simulink library "CDS_PARTS"  (Simulink 7.2)
settings: Solver=ode45  SolverMode=SingleTasking  StartTime=0.0  StopTime=10.0  RelTol=1e-3
undefined symbols (not defined in the file): dac, Subsystem
libraries: CDS_PARTS x5, simulink x2, cdsEXC x1, cdsEpicsBinIn x1, cdsEpicsIn x1, cdsEpicsMomentary x1, cdsEpicsOut x1, cdsRemoteIntlk x1, cdsEzCaRead x1, cdsEzCaWrite x1, cdsFiltCtrl x1, cdsFilt x1
settings Model: Creator=aivanov  LastModifiedBy=rolf  ExtModeAutoUpdateStatusClock=off

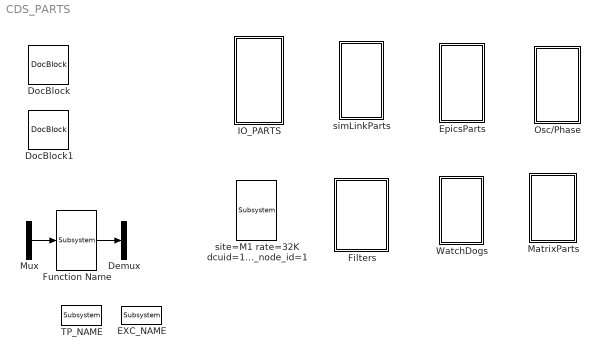
== system CDS_PARTS ==
  Demux : Demux  Outputs=2
  DocBlock : simulink/Model-Wide Utilities/DocBlock  Tag=Overview  SystemSampleTime=-1  DocumentType=Text
      settings: AttributesFormatString=%<Tag>
  DocBlock1 : simulink/Model-Wide Utilities/DocBlock  Tag=SW Install  SystemSampleTime=-1  DocumentType=Text
      settings: AttributesFormatString=%<Tag>
  EXC_NAME : cdsEXC/Subsystem  Tag=Excitation  SystemSampleTime=-1
      settings: AttributesFormatString=%<Tag>
  EpicsParts : Subsystem
  Filters : Subsystem
  Function Name : cdsFunctionCall/Subsystem  Tag=cdsFunctionCall  Description=|  SystemSampleTime=-1
      | Allows to make a call to external C function from the front-end code.                                                                                        
      | User needs to use a Mux and a Demux to proved N number of inputs and M number of outputs to an external function.                                            
      | Function "Foo()" code needs to be put in a file Foo.c in advLigo/src/fe/<model> directory.                                                                   
      |                                                                                                                                                              
      | Mon Apr  6 15:31:59 PDT 2009, by aivanov                                                                                                                     
      | It is possible now to put the same code you would normally keep in a file right here in this Description text box. The very first line needs to be 8 symbols:
      | //inline                                                                                                                                                     
      |                                                                                                                                                              
      | Then function definition follows exactly like you would put it in a file mentioned above.
      settings: AttributesFormatString=%<Tag>
  IO_PARTS : Subsystem
  MatrixParts : Subsystem
  Mux : Mux  Inputs=2
  Osc/Phase : Subsystem
  TP_NAME : cdsTP/Subsystem  Tag=Test Point  SystemSampleTime=-1
      settings: AttributesFormatString=%<Tag>
  WatchDogs : Subsystem
  simLinkParts : Subsystem
  site=M1 rate=32K dcuid=10 gds_node_id=1 : cdsParameters/Subsystem  Tag=cdsParameters  Description=|  SystemSampleTime=-1
      | Purpose:                                                                                                                                                                                                                                
      | Provide system parameters to the FE code generator to properly configure the generated EPICS names, rep rate of the FE controller, and the Data Acquisition node ID for proper storage of data from this FE controller.                 
      |                                                                                                                                                                                                                                         
      | Useage:                                                                                                                                                                                                                                 
      | The part NAME field is used to identify the FE parameters. It must be of the form:                                                                                                                                                      
      | site=                                                                                                                                                                                                                                   
      | rate=                                                                                                                                                                                                                                   
      | dcuid=                                                                                                                                                                                                                                  
      |                                                                                                                                                                                                                                         
      | Where:                                                                                                                                                                                                                                  
      | site= argument may be H1, H2, L1, M1, G1, either as a single argument or multiple, for example site=H1,H2. These are the only names allowed. These will become the first two characters of all EPICS and signal names (for example G1:).
      |                                                                                                                                                                                                                                         
      | rate= may be 2K, 16K, 32K, or 64K                                                                                                                                                                                                       
      |                                                                                                                                                                                                                                         
      | dcuid= is site specific ie it must be unique at each site.
      settings: AttributesFormatString=%<Tag>
  wires:
  Function Name/1 -> Demux/1
  Mux/1 -> Function Name/1

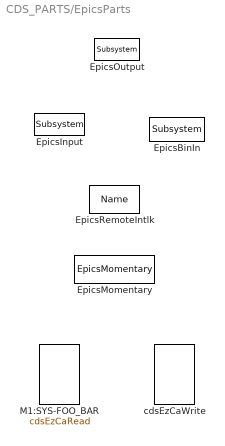
== system CDS_PARTS/EpicsParts ==
  EpicsBinIn : cdsEpicsBinIn/Subsystem  Tag=cdsEpicsBinIn  Description=|  SystemSampleTime=-1
      | Purpose:                                                                            
      | Create an EPICS binary (0 or 1) input channel to the FE realtime controls.          
      |                                                                                     
      | Operation:                                                                          
      | Outputs value from an EPICS ai record. Value is binary input (bi Epics record type).
      |                                                                                     
      | Usage:                                                                              
      | Name the part with the desired EPICS channel name.
      settings: AttributesFormatString=%<Tag>
  EpicsInput : cdsEpicsIn/Subsystem  Tag=cdsEpicsIn  Description=|  SystemSampleTime=-1
      | Purpose:                                                                              
      | Create an EPICS input channel connection to the FE realtime controls.                 
      |                                                                                       
      | Operation:                                                                            
      | Outputs value from an EPICS ai record. Value is floating point with a precision of 3..
      |                                                                                       
      | Usage:                                                                                
      | Name the part with the desired EPICS channel name.
      settings: AttributesFormatString=%<Tag>
  EpicsMomentary : cdsEpicsMomentary/EpicsMomentary  Tag=cdsEpicsMomentary  SystemSampleTime=-1
      settings: AttributesFormatString=%<Tag>
  EpicsOutput : cdsEpicsOut/Subsystem  Tag=cdsEpicsOutput  Description=|  SystemSampleTime=-1
      | Purpose:                                          
      | Output a FE signal to an EPICS channel.           
      |                                                   
      | Operation:                                        
      | Takes input value and passes it to EPICS record.  
      |                                                   
      | Usage:                                            
      | Name the part with the desired EPICS rrecord name.
      settings: AttributesFormatString=%<Tag>
  EpicsRemoteIntlk : cdsRemoteIntlk/Name  Tag=cdsRemoteIntlk  Description=|  SystemSampleTime=-1
      | Purpose:                                                                                                                                                                                                                                                                            
      | Used to turn off a switch in another subsystem using EPICS channel access. Typically, this is used as a remote interlock function.                                                                                                                                                  
      |                                                                                                                                                                                                                                                                                     
      | Operation:                                                                                                                                                                                                                                                                          
      | If input is zero, sends a zero to the specified EPICS channel name. Any other input value results in a NOOP. Input must be an integer.                                                                                                                                              
      |                                                                                                                                                                                                                                                                                     
      | Usage: Give the name of the EPICS channel to be written to, including the subsystem. For example: SEI-HMY_ACT_SW. This function will also produce a local EPICS variable for monitoring. For example, the above would result in a local EPICS variable of IFO:SUBSYS-SEI_HMY_ACT_SW.
      settings: AttributesFormatString=%<Tag>
  M1:SYS-FOO_BAR : cdsEzCaRead/cdsEzCaRead  Tag=cdsEzCaRead  Description=|  SystemSampleTime=-1
      | Purpose:                                                       
      | Used to input an Epics signal.                                 
      |                                                                
      | Operation:                                                     
      | Using ezcaread() function to get Epics input from a remote IOC.
      |                                                                
      | Usage:                                                         
      | Give the name of the EPICS channel to be read.
      settings: AttributesFormatString=%<Tag>
  cdsEzCaWrite : cdsEzCaWrite/cdsEzCaWrite  Tag=cdsEzCaWrite  Description=|  SystemSampleTime=-1
      | Purpose:                                    
      | Output Epics channel.                       
      |                                             
      | Operation:                                  
      | Using ezcawrite() output an Epics channel.  
      |                                             
      | Usage:                                      
      | Give the name of the EPICS channel to write.
      settings: AttributesFormatString=%<Tag>

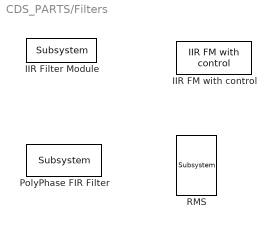
== system CDS_PARTS/Filters ==
  IIR FM with control : cdsFiltCtrl/IIR FM with control  Tag=cdsFiltCtrl  Description=|  SystemSampleTime=-1
      | cdsFiltCntrl is the standard IIR filter module (exactly the same as cdsFilt) but with added control data output 'Ctrl'. Filter module digital signal output appears on the first output, which is called 'Val'. 'Ctrl' output has a bit pattern encoding the state of filter's on/off switches (FM1 through FM10). The bit values are:
      |                                                                                                                                                                                                                                                                                                                                       
      | module 	hex	dec                                                                                                                                                                                                                                                                                                                       
      | -----------------------                                                                                                                                                                                                                                                                                                               
      | FM1	0x20                    32                                                                                                                                                                                                                                                                                                        
      | FM2	0x80                     128                                                                                                                                                                                                                                                                                                      
      | FM3	0x200                   512                                                                                                                                                                                                                                                                                                       
      | FM4	0x800                   2048                                                                                                                                                                                                                                                                                                      
      | FM5	0x2000                 8192                                                                                                                                                                                                                                                                                                       
      | FM6	0x8000                 32768                                                                                                                                                                                                                                                                                                      
      | FM7	0x20000                131072                                                                                                                                                                                                                                                                                                     
      | FM8	0x80000                 524288                                                                                                                                                                                                                                                                                                    
      | FM9	0x200000               2097152                                                                                                                                                                                                                                                                                                    
      | FM10	0x800000               8388608                                                                                                                                                                                                                                                                                                   
      |                                                                                                                                                                                                                                                                                                                                       
      | This bit data can be used to drive some other switches or it can be output using a binary I/O module.
      settings: AttributesFormatString=%<Tag>
  IIR Filter Module : cdsFilt/Subsystem  Tag=cdsFilt  Description=|  SystemSampleTime=-1
      | Purpose:                                                                                                                                                                                                                                  
      | Standard CDS IIR filter module.                                                                                                                                                                                                           
      |                                                                                                                                                                                                                                           
      | Operation:                                                                                                                                                                                                                                
      | Consists of 10 second order section IIR filters, plus a ramped gain stage. In FE code, also provides pre-defined test points and excitation channel inputs. The filter coefficients are defined in the LIGO system using the 'foton' tool.
      |                                                                                                                                                                                                                                           
      | Usage:                                                                                                                                                                                                                                    
      | Name the part with the desired filter module name.
      settings: AttributesFormatString=%<Tag>
  PolyPhase FIR Filter : cdsPPFIR/Subsystem  Tag=cdsPPFIR  Description=|  SystemSampleTime=-1
      | Purpose:                                                                                                    
      | Provide a Polyphase FIR filter algorithm. This part is typically only used in HEPI or other seismic systems.
      settings: AttributesFormatString=%<Tag>
  RMS : cdsRms/Subsystem  Tag=cdsRms  Description=|  SystemSampleTime=-1
      | Purpose:
      | Calculate an RMS based on the input signal.
      settings: AttributesFormatString=%<Tag>

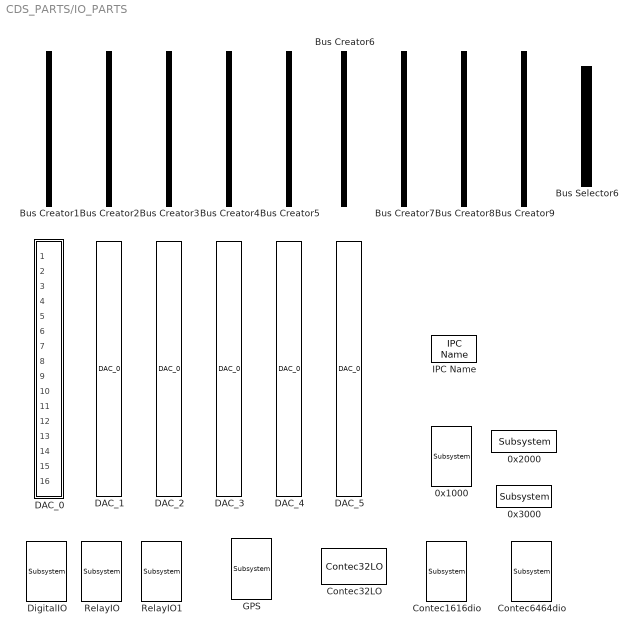
== system CDS_PARTS/IO_PARTS ==
  0x1000 : cdsRfmIO/Subsystem  Tag=cdsRfmIO  Description=VMIC5565 Reflective Memory read/write  SystemSampleTime=-1
      settings: AttributesFormatString=%<Tag>
  0x2000 : cdsIPC/Subsystem  Tag=cdsIPC  Description=Inter-process communication through /rtl_epics_ipc shared memory  SystemSampleTime=-1
      settings: AttributesFormatString=%<Tag>
  0x3000 : cdsIPCS/Subsystem  Tag=cdsIPCS  SystemSampleTime=-1
      settings: AttributesFormatString=%<Tag>
  Bus Creator1 : BusCreator  Tag=adc_0  Description=|  Inputs='adc_0_0','adc_0_1','adc_0_2','adc_0_3','adc_0_4','adc_0_5','adc_0_6','adc_0_7','adc_0_8','adc_0_9','adc_0_10','adc_0_11','adc_0_12','adc_0_13','adc_0_14','adc_0_15','adc_0_16','adc_0_17','adc_0_18','adc_0_19','adc_0_20','adc_0_21','adc_0_22','adc_0_23','adc_0_24','adc_0_25','adc_0_26','adc_0_27','adc_0_28','adc_0_29','adc_0_30','adc_0_31'
      | ADC0      
      | card_num=0
      settings: AttributesFormatString=%<Description>
  Bus Creator2 : BusCreator  Description=|  Inputs='adc_1_0','adc_1_1','adc_1_2','adc_1_3','adc_1_4','adc_1_5','adc_1_6','adc_1_7','adc_1_8','adc_1_9','adc_1_10','adc_1_11','adc_1_12','adc_1_13','adc_1_14','adc_1_15','adc_1_16','adc_1_17','adc_1_18','adc_1_19','adc_1_20','adc_1_21','adc_1_22','adc_1_23','adc_1_24','adc_1_25','adc_1_26','adc_1_27','adc_1_28','adc_1_29','adc_1_30','adc_1_31'
      | ADC1      
      | card_num=1
      settings: AttributesFormatString=%<Description>
  Bus Creator3 : BusCreator  Description=|  Inputs='adc_2_0','adc_2_1','adc_2_2','adc_2_3','adc_2_4','adc_2_5','adc_2_6','adc_2_7','adc_2_8','adc_2_9','adc_2_10','adc_2_11','adc_2_12','adc_2_13','adc_2_14','adc_2_15','adc_2_16','adc_2_17','adc_2_18','adc_2_19','adc_2_20','adc_2_21','adc_2_22','adc_2_23','adc_2_24','adc_2_25','adc_2_26','adc_2_27','adc_2_28','adc_2_29','adc_2_30','adc_2_31'
      | ADC2      
      | card_num=2
      settings: AttributesFormatString=%<Description>
  Bus Creator4 : BusCreator  Description=|  Inputs='adc_3_0','adc_3_1','adc_3_2','adc_3_3','adc_3_4','adc_3_5','adc_3_6','adc_3_7','adc_3_8','adc_3_9','adc_3_10','adc_3_11','adc_3_12','adc_3_13','adc_3_14','adc_3_15','adc_3_16','adc_3_17','adc_3_18','adc_3_19','adc_3_20','adc_3_21','adc_3_22','adc_3_23','adc_3_24','adc_3_25','adc_3_26','adc_3_27','adc_3_28','adc_3_29','adc_3_30','adc_3_31'
      | ADC3      
      | card_num=3
      settings: AttributesFormatString=%<Description>
  Bus Creator5 : BusCreator  Description=|  Inputs='adc_4_0','adc_4_1','adc_4_2','adc_4_3','adc_4_4','adc_4_5','adc_4_6','adc_4_7','adc_4_8','adc_4_9','adc_4_10','adc_4_11','adc_4_12','adc_4_13','adc_4_14','adc_4_15','adc_4_16','adc_4_17','adc_4_18','adc_4_19','adc_4_20','adc_4_21','adc_4_22','adc_4_23','adc_4_24','adc_4_25','adc_4_26','adc_4_27','adc_4_28','adc_4_29','adc_4_30','adc_4_31'
      | ADC4      
      | card_num=4
      settings: AttributesFormatString=%<Description>
  Bus Creator6 : BusCreator  Description=|  Inputs='adc_5_0','adc_5_1','adc_5_2','adc_5_3','adc_5_4','adc_5_5','adc_5_6','adc_5_7','adc_5_8','adc_5_9','adc_5_10','adc_5_11','adc_5_12','adc_5_13','adc_5_14','adc_5_15','adc_5_16','adc_5_17','adc_5_18','adc_5_19','adc_5_20','adc_5_21','adc_5_22','adc_5_23','adc_5_24','adc_5_25','adc_5_26','adc_5_27','adc_5_28','adc_5_29','adc_5_30','adc_5_31'
      | ADC5      
      | card_num=5
      settings: AttributesFormatString=%<Description>
  Bus Creator7 : BusCreator  Description=|  Inputs='adc_6_0','adc_6_1','adc_6_2','adc_6_3','adc_6_4','adc_6_5','adc_6_6','adc_6_7','adc_6_8','adc_6_9','adc_6_10','adc_6_11','adc_6_12','adc_6_13','adc_6_14','adc_6_15','adc_6_16','adc_6_17','adc_6_18','adc_6_19','adc_6_20','adc_6_21','adc_6_22','adc_6_23','adc_6_24','adc_6_25','adc_6_26','adc_6_27','adc_6_28','adc_6_29','adc_6_30','adc_6_31'
      | ADC6      
      | card_num=6
      settings: AttributesFormatString=%<Description>
  Bus Creator8 : BusCreator  Description=|  Inputs='adc_7_0','adc_7_1','adc_7_2','adc_7_3','adc_7_4','adc_7_5','adc_7_6','adc_7_7','adc_7_8','adc_7_9','adc_7_10','adc_7_11','adc_7_12','adc_7_13','adc_7_14','adc_7_15','adc_7_16','adc_7_17','adc_7_18','adc_7_19','adc_7_20','adc_7_21','adc_7_22','adc_7_23','adc_7_24','adc_7_25','adc_7_26','adc_7_27','adc_7_28','adc_7_29','adc_7_30','adc_7_31'
      | ADC7      
      | card_num=7
      settings: AttributesFormatString=%<Description>
  Bus Creator9 : BusCreator  Description=|  Inputs='adc_8_0','adc_8_1','adc_8_2','adc_8_3','adc_8_4','adc_8_5','adc_8_6','adc_8_7','adc_8_8','adc_8_9','adc_8_10','adc_8_11','adc_8_12','adc_8_13','adc_8_14','adc_8_15','adc_8_16','adc_8_17','adc_8_18','adc_8_19','adc_8_20','adc_8_21','adc_8_22','adc_8_23','adc_8_24','adc_8_25','adc_8_26','adc_8_27','adc_8_28','adc_8_29','adc_8_30','adc_8_31'
      | ADC8      
      | card_num=8
      settings: AttributesFormatString=%<Description>
  Bus Selector6 : BusSelector  Description=ADC Selector  OutputSignals=adc_0_0,adc_0_1
      settings: AttributesFormatString=%<Description>
  Contec1616dio : cdsContec1616DIO/Subsystem  Tag=cdsCDIO1616  SystemSampleTime=-1
      settings: AttributesFormatString=%<Tag>
  Contec32LO : cdsCDO32/Contec32LO  Tag=cdsCDO32  Description=Contec32 bit binary output module driver  SystemSampleTime=-1
      settings: AttributesFormatString=%<Tag>
  Contec6464dio : cdsContec6464DIO/Subsystem  Tag=cdsDIO6464  SystemSampleTime=-1
      settings: AttributesFormatString=%<Tag>
  DAC_0 : Subsystem  Description=card_num=0  AncestorBlock=dac/Subsystem
      settings: AttributesFormatString=%<Description>
  DAC_1 : CDS_PARTS/IO_PARTS/DAC_0  Description=card_num=1  SystemSampleTime=-1
      settings: AttributesFormatString=%<Description>
  DAC_2 : CDS_PARTS/IO_PARTS/DAC_0  Description=card_num=2  SystemSampleTime=-1
      settings: AttributesFormatString=%<Description>
  DAC_3 : CDS_PARTS/IO_PARTS/DAC_0  Description=card_num=3  SystemSampleTime=-1
      settings: AttributesFormatString=%<Description>
  DAC_4 : CDS_PARTS/IO_PARTS/DAC_0  Description=card_num=4  SystemSampleTime=-1
      settings: AttributesFormatString=%<Description>
  DAC_5 : CDS_PARTS/IO_PARTS/DAC_0  Description=card_num=5  SystemSampleTime=-1
      settings: AttributesFormatString=%<Description>
  DigitalIO : cdsDio/Subsystem  Tag=cdsDio  Description=|  SystemSampleTime=-1
      | support for 8 bit input 8 bit output DIO PCI card
      | ACCESS I/O Products model DIO-24D
      settings: AttributesFormatString=%<Tag>
  GPS : cdsGps/Subsystem  Tag=cdsGps  Description=|  SystemSampleTime=-1
      | Symmetricom BC635PCI-U GPS card input                                 
      | This block outputs current time as sampled using the card.            
      | full -- complete UNIX seconds, and fractional part correct up to 100ns
      | s    -- integer UNIX seconds (no fraction)                            
      | us  -- fractional part                                                
      | ns  -- nanoseconds part
  IPC Name : IPCx/IPC Name  Tag=cdsIPCx  Description=Inter-process communication through /rtl_epics_ipc shared memory  SystemSampleTime=-1
      settings: AttributesFormatString=%<Tag>
  RelayIO : cdsRio/Subsystem  Tag=cdsRio  Description=PCI IIRO 8 relay output and isolated input module  SystemSampleTime=-1
      settings: AttributesFormatString=%<Tag>
  RelayIO1 : cdsRio1/Subsystem  Tag=cdsRio1  Description=PCI IIRO 16 channel relay ourput and isolated input module  SystemSampleTime=-1
      settings: AttributesFormatString=%<Tag>

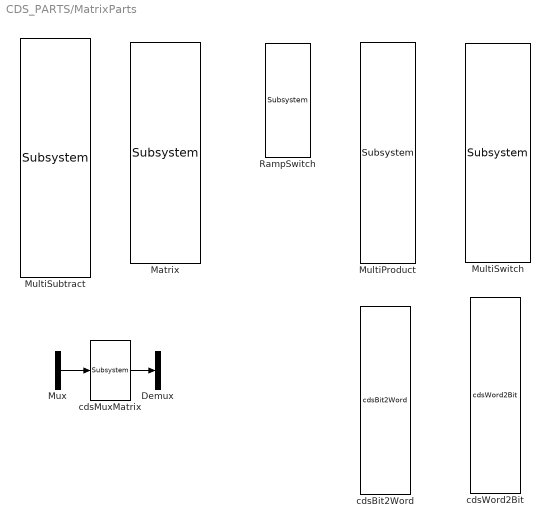
== system CDS_PARTS/MatrixParts ==
  Demux : Demux  Outputs=2
  Matrix : cdsMatrix/Subsystem  Tag=Matrix  Description=|  SystemSampleTime=-1
      | Purpose:                                                                 
      | Provide a matrix multiplication function for up to 8 input and 8 outputs.
      settings: AttributesFormatString=%<Tag>
  MultiProduct : cdsProduct/Subsystem  Tag=cdsProduct  Description=|  SystemSampleTime=-1
      | Purpose:                                                                                                                                                                      
      | Multiply 8 inputs by a common gain factor.                                                                                                                                    
      |                                                                                                                                                                               
      | Operation:                                                                                                                                                                    
      | Generates two epics records: partName and partName_TRAMP. All eight inputs are multiplied by the EPICS partName input, ramped over a duration (in seconds) of the TRAMP input.
      settings: AttributesFormatString=%<Tag>
  MultiSubtract : cdsSubtract8/Subsystem  Tag=cdsSubtract8  Description=|  SystemSampleTime=-1
      | Purpose:
      | Subtract pairs of 16 inputs.
      settings: AttributesFormatString=%<Tag>
  MultiSwitch : cdsSwitch1/Subsystem  Tag=cdsSwitch1  Description=Switch  SystemSampleTime=-1
      settings: AttributesFormatString=%<Tag>
  Mux : Mux  Inputs=2
  RampSwitch : cdsRampSwitch/Subsystem  Tag=cdsRampSwitch  Description=Ramp Switch  SystemSampleTime=-1
      settings: AttributesFormatString=%<Tag>
  cdsBit2Word : cdsBit2Word/cdsBit2Word  Tag=cdsBit2Word  Description=Forms single 16 bit integer from 16 0/1 inputs.  SystemSampleTime=-1
      settings: AttributesFormatString=%<Tag>
  cdsMuxMatrix : cdsMuxMatrix/Subsystem  Tag=cdsMuxMatrix  Description=Any size matrix. Inputs and outputs must be connected using Mux and Demux parts.  SystemSampleTime=-1
      settings: AttributesFormatString=%<Tag>
  cdsWord2Bit : cdsWord2Bit/cdsWord2Bit  Tag=cdsWord2Bit  Description=Generate 16 0/1 outputs from single 16-bit integer input  SystemSampleTime=-1
      settings: AttributesFormatString=cdsWord2Bit
  wires:
  Mux/1 -> cdsMuxMatrix/1
  cdsMuxMatrix/1 -> Demux/1

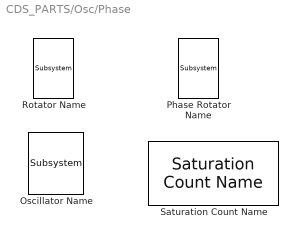
== system CDS_PARTS/Osc/Phase ==
  Oscillator Name : cdsOsc/Subsystem  Tag=cdsOsc  Description=Oscillator  SystemSampleTime=-1
      settings: AttributesFormatString=%<Tag>
  Phase Rotator Name : cdsPhase/Subsystem  Tag=cdsPhase  Description=Phase Rotator  SystemSampleTime=-1
      settings: AttributesFormatString=%<Tag>
  Rotator Name : cdsWfsPhase/Subsystem  Tag=cdsWfsPhase  Description=WFS Phase Rotator  SystemSampleTime=-1
      settings: AttributesFormatString=%<Tag>
  Saturation Count Name : cdsSatCount/Saturation Count Name  Tag=cdsSatCount  Description=Saturation count  SystemSampleTime=-1
      settings: AttributesFormatString=%<Tag>

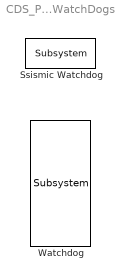
== system CDS_PARTS/WatchDogs ==
  Ssismic Watchdog : cdsSusWd/Subsystem  Tag=cdsSusWd  Description=Sus Watchdog  SystemSampleTime=-1
      settings: AttributesFormatString=%<Tag>
  Watchdog : cdsWD/Subsystem  Description=cdsWD  SystemSampleTime=-1
      settings: AttributesFormatString=%<Description>

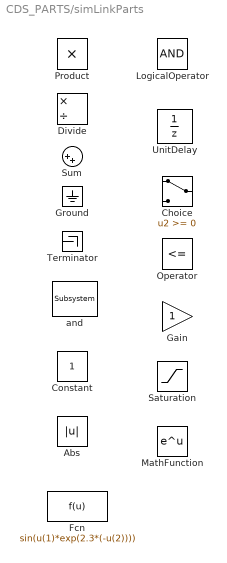
== system CDS_PARTS/simLinkParts ==
  Abs : Abs
  Choice : Switch
  Constant : Constant  OutDataType=sfix(16)  OutScaling=2^0
  Divide : Product  Inputs=*/  OutDataType=sfix(16)  OutScaling=2^-10
  Fcn : Fcn  Expr=sin(u(1)*exp(2.3*(-u(2))))
  Gain : Gain  ParameterDataType=sfix(16)  ParameterScaling=2^0  OutDataType=sfix(16)  OutScaling=2^0
  Ground : Ground
  LogicalOperator : Logic  AllPortsSameDT=off  OutDataTypeMode=boolean  OutDataTypeStr=boolean
  MathFunction : Math  OutDataType=sfix(16)  OutScaling=2^0  SaturateOnIntegerOverflow=on
  Operator : RelationalOperator  Operator=<=  LogicOutDataTypeMode=boolean  OutDataTypeStr=boolean
  Product : Product  OutDataType=sfix(16)  OutScaling=2^0  RndMeth=Zero
  Saturation : Saturate
  Sum : Sum  Inputs=|++  OutDataType=sfix(16)  OutScaling=2^0
  Terminator : Terminator
  UnitDelay : UnitDelay
  and : cdsBitwise/Subsystem  Tag=cdsBitwise  SystemSampleTime=-1
      settings: AttributesFormatString=%<Tag>

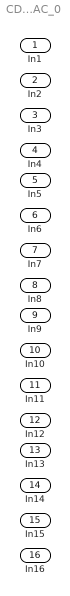
== system CDS_PARTS/IO_PARTS/DAC_0 ==
  In1 : Inport  OutDataType=sfix(16)  OutScaling=2^0
  In2 : Inport  Port=2  OutDataType=sfix(16)  OutScaling=2^0
  In3 : Inport  Port=3  OutDataType=sfix(16)  OutScaling=2^0
  In4 : Inport  Port=4  OutDataType=sfix(16)  OutScaling=2^0
  In5 : Inport  Port=5  OutDataType=sfix(16)  OutScaling=2^0
  In6 : Inport  Port=6  OutDataType=sfix(16)  OutScaling=2^0
  In7 : Inport  Port=7  OutDataType=sfix(16)  OutScaling=2^0
  In8 : Inport  Port=8  OutDataType=sfix(16)  OutScaling=2^0
  In9 : Inport  Port=9  OutDataType=sfix(16)  OutScaling=2^0
  In10 : Inport  Port=10  OutDataType=sfix(16)  OutScaling=2^0
  In11 : Inport  Port=11  OutDataType=sfix(16)  OutScaling=2^0
  In12 : Inport  Port=12  OutDataType=sfix(16)  OutScaling=2^0
  In13 : Inport  Port=13  OutDataType=sfix(16)  OutScaling=2^0
  In14 : Inport  Port=14  OutDataType=sfix(16)  OutScaling=2^0
  In15 : Inport  Port=15  OutDataType=sfix(16)  OutScaling=2^0
  In16 : Inport  Port=16  OutDataType=sfix(16)  OutScaling=2^0
